simulink model "AC_Test"  (R2021b)
settings: Solver=VariableStepAuto  StartTime=0.0  StopTime=1  RelTol=1e-3
undefined symbols (not defined in the file): ac
libraries: fl_lib x132, nesl_utility x4
settings Model: Creator=김웅지  LastModifiedBy=김웅지

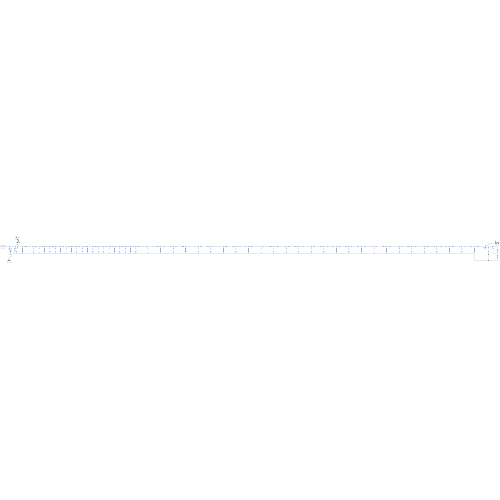
[thumbnail: Simulink's stored preview of the top-level diagram]
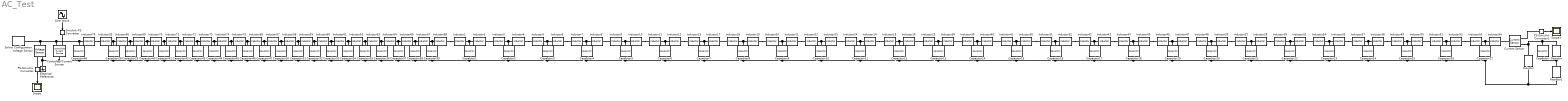
== system AC_Test ==
  Capacitor : fl_lib/Electrical/Electrical Elements/Capacitor  c=ac.rad.Cm1 F  r=1e-15 Ohm  g=0 1/Ohm  i_specify=off  i_priority=None  i=0 A  i_nominal_specify=off  i_nominal_unit=A  i_nominal_value=1  v_specify=off  v_priority=None  v=0 V  v_nominal_specify=off  v_nominal_unit=V  v_nominal_value=1  vc_specify=off  vc_priority=High  vc=0 V  vc_nominal_specify=off  vc_nominal_unit=V  vc_nominal_value=1
  Capacitor1 : fl_lib/Electrical/Electrical Elements/Capacitor  c=ac.ho.C(1) F  r=1e-15 Ohm  g=0 1/Ohm  i_specify=off  i_priority=None  i=0 A  i_nominal_specify=off  i_nominal_unit=A  i_nominal_value=1  v_specify=off  v_priority=None  v=0 V  v_nominal_specify=off  v_nominal_unit=V  v_nominal_value=1  vc_specify=off  vc_priority=High  vc=0 V  vc_nominal_specify=off  vc_nominal_unit=V  vc_nominal_value=1
  Capacitor10 : fl_lib/Electrical/Electrical Elements/Capacitor  c=ac.ho.C(10) F  r=1e-15 Ohm  g=0 1/Ohm  i_specify=off  i_priority=None  i=0 A  i_nominal_specify=off  i_nominal_unit=A  i_nominal_value=1  v_specify=off  v_priority=None  v=0 V  v_nominal_specify=off  v_nominal_unit=V  v_nominal_value=1  vc_specify=off  vc_priority=High  vc=0 V  vc_nominal_specify=off  vc_nominal_unit=V  vc_nominal_value=1
  Capacitor11 : fl_lib/Electrical/Electrical Elements/Capacitor  c=ac.ho.C(11) F  r=1e-15 Ohm  g=0 1/Ohm  i_specify=off  i_priority=None  i=0 A  i_nominal_specify=off  i_nominal_unit=A  i_nominal_value=1  v_specify=off  v_priority=None  v=0 V  v_nominal_specify=off  v_nominal_unit=V  v_nominal_value=1  vc_specify=off  vc_priority=High  vc=0 V  vc_nominal_specify=off  vc_nominal_unit=V  vc_nominal_value=1
  Capacitor12 : fl_lib/Electrical/Electrical Elements/Capacitor  c=ac.ho.C(12) F  r=1e-15 Ohm  g=0 1/Ohm  i_specify=off  i_priority=None  i=0 A  i_nominal_specify=off  i_nominal_unit=A  i_nominal_value=1  v_specify=off  v_priority=None  v=0 V  v_nominal_specify=off  v_nominal_unit=V  v_nominal_value=1  vc_specify=off  vc_priority=High  vc=0 V  vc_nominal_specify=off  vc_nominal_unit=V  vc_nominal_value=1
  Capacitor13 : fl_lib/Electrical/Electrical Elements/Capacitor  c=ac.ho.C(13) F  r=1e-15 Ohm  g=0 1/Ohm  i_specify=off  i_priority=None  i=0 A  i_nominal_specify=off  i_nominal_unit=A  i_nominal_value=1  v_specify=off  v_priority=None  v=0 V  v_nominal_specify=off  v_nominal_unit=V  v_nominal_value=1  vc_specify=off  vc_priority=High  vc=0 V  vc_nominal_specify=off  vc_nominal_unit=V  vc_nominal_value=1
  Capacitor14 : fl_lib/Electrical/Electrical Elements/Capacitor  c=ac.ho.C(14) F  r=1e-15 Ohm  g=0 1/Ohm  i_specify=off  i_priority=None  i=0 A  i_nominal_specify=off  i_nominal_unit=A  i_nominal_value=1  v_specify=off  v_priority=None  v=0 V  v_nominal_specify=off  v_nominal_unit=V  v_nominal_value=1  vc_specify=off  vc_priority=High  vc=0 V  vc_nominal_specify=off  vc_nominal_unit=V  vc_nominal_value=1
  Capacitor15 : fl_lib/Electrical/Electrical Elements/Capacitor  c=ac.ho.C(15) F  r=1e-15 Ohm  g=0 1/Ohm  i_specify=off  i_priority=None  i=0 A  i_nominal_specify=off  i_nominal_unit=A  i_nominal_value=1  v_specify=off  v_priority=None  v=0 V  v_nominal_specify=off  v_nominal_unit=V  v_nominal_value=1  vc_specify=off  vc_priority=High  vc=0 V  vc_nominal_specify=off  vc_nominal_unit=V  vc_nominal_value=1
  Capacitor16 : fl_lib/Electrical/Electrical Elements/Capacitor  c=ac.ho.C(16) F  r=1e-15 Ohm  g=0 1/Ohm  i_specify=off  i_priority=None  i=0 A  i_nominal_specify=off  i_nominal_unit=A  i_nominal_value=1  v_specify=off  v_priority=None  v=0 V  v_nominal_specify=off  v_nominal_unit=V  v_nominal_value=1  vc_specify=off  vc_priority=High  vc=0 V  vc_nominal_specify=off  vc_nominal_unit=V  vc_nominal_value=1
  Capacitor17 : fl_lib/Electrical/Electrical Elements/Capacitor  c=ac.ho.C(17) F  r=1e-15 Ohm  g=0 1/Ohm  i_specify=off  i_priority=None  i=0 A  i_nominal_specify=off  i_nominal_unit=A  i_nominal_value=1  v_specify=off  v_priority=None  v=0 V  v_nominal_specify=off  v_nominal_unit=V  v_nominal_value=1  vc_specify=off  vc_priority=High  vc=0 V  vc_nominal_specify=off  vc_nominal_unit=V  vc_nominal_value=1
  Capacitor18 : fl_lib/Electrical/Electrical Elements/Capacitor  c=ac.ho.C(18) F  r=1e-15 Ohm  g=0 1/Ohm  i_specify=off  i_priority=None  i=0 A  i_nominal_specify=off  i_nominal_unit=A  i_nominal_value=1  v_specify=off  v_priority=None  v=0 V  v_nominal_specify=off  v_nominal_unit=V  v_nominal_value=1  vc_specify=off  vc_priority=High  vc=0 V  vc_nominal_specify=off  vc_nominal_unit=V  vc_nominal_value=1
  Capacitor19 : fl_lib/Electrical/Electrical Elements/Capacitor  c=ac.ho.C(19) F  r=1e-15 Ohm  g=0 1/Ohm  i_specify=off  i_priority=None  i=0 A  i_nominal_specify=off  i_nominal_unit=A  i_nominal_value=1  v_specify=off  v_priority=None  v=0 V  v_nominal_specify=off  v_nominal_unit=V  v_nominal_value=1  vc_specify=off  vc_priority=High  vc=0 V  vc_nominal_specify=off  vc_nominal_unit=V  vc_nominal_value=1
  Capacitor2 : fl_lib/Electrical/Electrical Elements/Capacitor  c=ac.ho.C(2) F  r=1e-15 Ohm  g=0 1/Ohm  i_specify=off  i_priority=None  i=0 A  i_nominal_specify=off  i_nominal_unit=A  i_nominal_value=1  v_specify=off  v_priority=None  v=0 V  v_nominal_specify=off  v_nominal_unit=V  v_nominal_value=1  vc_specify=off  vc_priority=High  vc=0 V  vc_nominal_specify=off  vc_nominal_unit=V  vc_nominal_value=1
  Capacitor20 : fl_lib/Electrical/Electrical Elements/Capacitor  c=ac.ho.C(20) F  r=1e-15 Ohm  g=0 1/Ohm  i_specify=off  i_priority=None  i=0 A  i_nominal_specify=off  i_nominal_unit=A  i_nominal_value=1  v_specify=off  v_priority=None  v=0 V  v_nominal_specify=off  v_nominal_unit=V  v_nominal_value=1  vc_specify=off  vc_priority=High  vc=0 V  vc_nominal_specify=off  vc_nominal_unit=V  vc_nominal_value=1
  Capacitor21 : fl_lib/Electrical/Electrical Elements/Capacitor  c=ac.ho.C(21) F  r=1e-15 Ohm  g=0 1/Ohm  i_specify=off  i_priority=None  i=0 A  i_nominal_specify=off  i_nominal_unit=A  i_nominal_value=1  v_specify=off  v_priority=None  v=0 V  v_nominal_specify=off  v_nominal_unit=V  v_nominal_value=1  vc_specify=off  vc_priority=High  vc=0 V  vc_nominal_specify=off  vc_nominal_unit=V  vc_nominal_value=1
  Capacitor22 : fl_lib/Electrical/Electrical Elements/Capacitor  c=ac.ho.C(22) F  r=1e-15 Ohm  g=0 1/Ohm  i_specify=off  i_priority=None  i=0 A  i_nominal_specify=off  i_nominal_unit=A  i_nominal_value=1  v_specify=off  v_priority=None  v=0 V  v_nominal_specify=off  v_nominal_unit=V  v_nominal_value=1  vc_specify=off  vc_priority=High  vc=0 V  vc_nominal_specify=off  vc_nominal_unit=V  vc_nominal_value=1
  Capacitor23 : fl_lib/Electrical/Electrical Elements/Capacitor  c=ac.ho.C(23) F  r=1e-15 Ohm  g=0 1/Ohm  i_specify=off  i_priority=None  i=0 A  i_nominal_specify=off  i_nominal_unit=A  i_nominal_value=1  v_specify=off  v_priority=None  v=0 V  v_nominal_specify=off  v_nominal_unit=V  v_nominal_value=1  vc_specify=off  vc_priority=High  vc=0 V  vc_nominal_specify=off  vc_nominal_unit=V  vc_nominal_value=1
  Capacitor24 : fl_lib/Electrical/Electrical Elements/Capacitor  c=ac.ho.C(24) F  r=1e-15 Ohm  g=0 1/Ohm  i_specify=off  i_priority=None  i=0 A  i_nominal_specify=off  i_nominal_unit=A  i_nominal_value=1  v_specify=off  v_priority=None  v=0 V  v_nominal_specify=off  v_nominal_unit=V  v_nominal_value=1  vc_specify=off  vc_priority=High  vc=0 V  vc_nominal_specify=off  vc_nominal_unit=V  vc_nominal_value=1
  Capacitor25 : fl_lib/Electrical/Electrical Elements/Capacitor  c=ac.ho.C(25) F  r=1e-15 Ohm  g=0 1/Ohm  i_specify=off  i_priority=None  i=0 A  i_nominal_specify=off  i_nominal_unit=A  i_nominal_value=1  v_specify=off  v_priority=None  v=0 V  v_nominal_specify=off  v_nominal_unit=V  v_nominal_value=1  vc_specify=off  vc_priority=High  vc=0 V  vc_nominal_specify=off  vc_nominal_unit=V  vc_nominal_value=1
  Capacitor26 : fl_lib/Electrical/Electrical Elements/Capacitor  c=ac.ho.C(26) F  r=1e-15 Ohm  g=0 1/Ohm  i_specify=off  i_priority=None  i=0 A  i_nominal_specify=off  i_nominal_unit=A  i_nominal_value=1  v_specify=off  v_priority=None  v=0 V  v_nominal_specify=off  v_nominal_unit=V  v_nominal_value=1  vc_specify=off  vc_priority=High  vc=0 V  vc_nominal_specify=off  vc_nominal_unit=V  vc_nominal_value=1
  Capacitor27 : fl_lib/Electrical/Electrical Elements/Capacitor  c=ac.ho.C(27) F  r=1e-15 Ohm  g=0 1/Ohm  i_specify=off  i_priority=None  i=0 A  i_nominal_specify=off  i_nominal_unit=A  i_nominal_value=1  v_specify=off  v_priority=None  v=0 V  v_nominal_specify=off  v_nominal_unit=V  v_nominal_value=1  vc_specify=off  vc_priority=High  vc=0 V  vc_nominal_specify=off  vc_nominal_unit=V  vc_nominal_value=1
  Capacitor{28..47} (20 alike) : fl_lib/Electrical/Electrical Elements/Capacitor  c=ac.ps.C F  r=1e-15 Ohm  g=0 1/Ohm  i_specify=off  i_priority=None  i=0 A  i_nominal_specify=off  i_nominal_unit=A  i_nominal_value=1  v_specify=off  v_priority=None  v=0 V  v_nominal_specify=off  v_nominal_unit=V  v_nominal_value=1  vc_specify=off  vc_priority=High  vc=0 V  vc_nominal_specify=off  vc_nominal_unit=V  vc_nominal_value=1
  Capacitor3 : fl_lib/Electrical/Electrical Elements/Capacitor  c=ac.ho.C(3) F  r=1e-15 Ohm  g=0 1/Ohm  i_specify=off  i_priority=None  i=0 A  i_nominal_specify=off  i_nominal_unit=A  i_nominal_value=1  v_specify=off  v_priority=None  v=0 V  v_nominal_specify=off  v_nominal_unit=V  v_nominal_value=1  vc_specify=off  vc_priority=High  vc=0 V  vc_nominal_specify=off  vc_nominal_unit=V  vc_nominal_value=1
  Capacitor4 : fl_lib/Electrical/Electrical Elements/Capacitor  c=ac.ho.C(4) F  r=1e-15 Ohm  g=0 1/Ohm  i_specify=off  i_priority=None  i=0 A  i_nominal_specify=off  i_nominal_unit=A  i_nominal_value=1  v_specify=off  v_priority=None  v=0 V  v_nominal_specify=off  v_nominal_unit=V  v_nominal_value=1  vc_specify=off  vc_priority=High  vc=0 V  vc_nominal_specify=off  vc_nominal_unit=V  vc_nominal_value=1
  Capacitor48 : fl_lib/Electrical/Electrical Elements/Capacitor  c=ac.co.C F  r=1e-15 Ohm  g=0 1/Ohm  i_specify=off  i_priority=None  i=0 A  i_nominal_specify=off  i_nominal_unit=A  i_nominal_value=1  v_specify=off  v_priority=None  v=0 V  v_nominal_specify=off  v_nominal_unit=V  v_nominal_value=1  vc_specify=off  vc_priority=High  vc=0 V  vc_nominal_specify=off  vc_nominal_unit=V  vc_nominal_value=1
  Capacitor5 : fl_lib/Electrical/Electrical Elements/Capacitor  c=ac.ho.C(5) F  r=1e-15 Ohm  g=0 1/Ohm  i_specify=off  i_priority=None  i=0 A  i_nominal_specify=off  i_nominal_unit=A  i_nominal_value=1  v_specify=off  v_priority=None  v=0 V  v_nominal_specify=off  v_nominal_unit=V  v_nominal_value=1  vc_specify=off  vc_priority=High  vc=0 V  vc_nominal_specify=off  vc_nominal_unit=V  vc_nominal_value=1
  Capacitor6 : fl_lib/Electrical/Electrical Elements/Capacitor  c=ac.ho.C(6) F  r=1e-15 Ohm  g=0 1/Ohm  i_specify=off  i_priority=None  i=0 A  i_nominal_specify=off  i_nominal_unit=A  i_nominal_value=1  v_specify=off  v_priority=None  v=0 V  v_nominal_specify=off  v_nominal_unit=V  v_nominal_value=1  vc_specify=off  vc_priority=High  vc=0 V  vc_nominal_specify=off  vc_nominal_unit=V  vc_nominal_value=1
  Capacitor7 : fl_lib/Electrical/Electrical Elements/Capacitor  c=ac.ho.C(7) F  r=1e-15 Ohm  g=0 1/Ohm  i_specify=off  i_priority=None  i=0 A  i_nominal_specify=off  i_nominal_unit=A  i_nominal_value=1  v_specify=off  v_priority=None  v=0 V  v_nominal_specify=off  v_nominal_unit=V  v_nominal_value=1  vc_specify=off  vc_priority=High  vc=0 V  vc_nominal_specify=off  vc_nominal_unit=V  vc_nominal_value=1
  Capacitor8 : fl_lib/Electrical/Electrical Elements/Capacitor  c=ac.ho.C(8) F  r=1e-15 Ohm  g=0 1/Ohm  i_specify=off  i_priority=None  i=0 A  i_nominal_specify=off  i_nominal_unit=A  i_nominal_value=1  v_specify=off  v_priority=None  v=0 V  v_nominal_specify=off  v_nominal_unit=V  v_nominal_value=1  vc_specify=off  vc_priority=High  vc=0 V  vc_nominal_specify=off  vc_nominal_unit=V  vc_nominal_value=1
  Capacitor9 : fl_lib/Electrical/Electrical Elements/Capacitor  c=ac.ho.C(9) F  r=1e-15 Ohm  g=0 1/Ohm  i_specify=off  i_priority=None  i=0 A  i_nominal_specify=off  i_nominal_unit=A  i_nominal_value=1  v_specify=off  v_priority=None  v=0 V  v_nominal_specify=off  v_nominal_unit=V  v_nominal_value=1  vc_specify=off  vc_priority=High  vc=0 V  vc_nominal_specify=off  vc_nominal_unit=V  vc_nominal_value=1
  Controlled Current Source : fl_lib/Electrical/Electrical Sources/Controlled Current Source
  Current Sensor : fl_lib/Electrical/Electrical Sensors/Current Sensor
  Electrical Reference : fl_lib/Electrical/Electrical Elements/Electrical Reference
  Inductor : fl_lib/Electrical/Electrical Elements/Inductor  l=ac.rad.Mm1 H  r=0 Ohm  g=1e-15 1/Ohm  i_specify=off  i_priority=None  i=0 A  i_nominal_specify=off  i_nominal_unit=A  i_nominal_value=1  v_specify=off  v_priority=None  v=0 V  v_nominal_specify=off  v_nominal_unit=V  v_nominal_value=1  i_L_specify=off  i_L_priority=High  i_L=0 A  i_L_nominal_specify=off  i_L_nominal_unit=A  i_L_nominal_value=1
  Inductor1 : fl_lib/Electrical/Electrical Elements/Inductor  l=ac.ho.L(1) H  r=0 Ohm  g=1e-15 1/Ohm  i_specify=off  i_priority=None  i=0 A  i_nominal_specify=off  i_nominal_unit=A  i_nominal_value=1  v_specify=off  v_priority=None  v=0 V  v_nominal_specify=off  v_nominal_unit=V  v_nominal_value=1  i_L_specify=off  i_L_priority=High  i_L=0 A  i_L_nominal_specify=off  i_L_nominal_unit=A  i_L_nominal_value=1
  Inductor10 : fl_lib/Electrical/Electrical Elements/Inductor  l=ac.ho.L(5) H  r=0 Ohm  g=1e-15 1/Ohm  i_specify=off  i_priority=None  i=0 A  i_nominal_specify=off  i_nominal_unit=A  i_nominal_value=1  v_specify=off  v_priority=None  v=0 V  v_nominal_specify=off  v_nominal_unit=V  v_nominal_value=1  i_L_specify=off  i_L_priority=High  i_L=0 A  i_L_nominal_specify=off  i_L_nominal_unit=A  i_L_nominal_value=1
  Inductor11 : fl_lib/Electrical/Electrical Elements/Inductor  l=ac.ho.L(6) H  r=0 Ohm  g=1e-15 1/Ohm  i_specify=off  i_priority=None  i=0 A  i_nominal_specify=off  i_nominal_unit=A  i_nominal_value=1  v_specify=off  v_priority=None  v=0 V  v_nominal_specify=off  v_nominal_unit=V  v_nominal_value=1  i_L_specify=off  i_L_priority=High  i_L=0 A  i_L_nominal_specify=off  i_L_nominal_unit=A  i_L_nominal_value=1
  Inductor12 : fl_lib/Electrical/Electrical Elements/Inductor  l=ac.ho.L(6) H  r=0 Ohm  g=1e-15 1/Ohm  i_specify=off  i_priority=None  i=0 A  i_nominal_specify=off  i_nominal_unit=A  i_nominal_value=1  v_specify=off  v_priority=None  v=0 V  v_nominal_specify=off  v_nominal_unit=V  v_nominal_value=1  i_L_specify=off  i_L_priority=High  i_L=0 A  i_L_nominal_specify=off  i_L_nominal_unit=A  i_L_nominal_value=1
  Inductor13 : fl_lib/Electrical/Electrical Elements/Inductor  l=ac.ho.L(7) H  r=0 Ohm  g=1e-15 1/Ohm  i_specify=off  i_priority=None  i=0 A  i_nominal_specify=off  i_nominal_unit=A  i_nominal_value=1  v_specify=off  v_priority=None  v=0 V  v_nominal_specify=off  v_nominal_unit=V  v_nominal_value=1  i_L_specify=off  i_L_priority=High  i_L=0 A  i_L_nominal_specify=off  i_L_nominal_unit=A  i_L_nominal_value=1
  Inductor14 : fl_lib/Electrical/Electrical Elements/Inductor  l=ac.ho.L(11) H  r=0 Ohm  g=1e-15 1/Ohm  i_specify=off  i_priority=None  i=0 A  i_nominal_specify=off  i_nominal_unit=A  i_nominal_value=1  v_specify=off  v_priority=None  v=0 V  v_nominal_specify=off  v_nominal_unit=V  v_nominal_value=1  i_L_specify=off  i_L_priority=High  i_L=0 A  i_L_nominal_specify=off  i_L_nominal_unit=A  i_L_nominal_value=1
  Inductor15 : fl_lib/Electrical/Electrical Elements/Inductor  l=ac.ho.L(12) H  r=0 Ohm  g=1e-15 1/Ohm  i_specify=off  i_priority=None  i=0 A  i_nominal_specify=off  i_nominal_unit=A  i_nominal_value=1  v_specify=off  v_priority=None  v=0 V  v_nominal_specify=off  v_nominal_unit=V  v_nominal_value=1  i_L_specify=off  i_L_priority=High  i_L=0 A  i_L_nominal_specify=off  i_L_nominal_unit=A  i_L_nominal_value=1
  Inductor16 : fl_lib/Electrical/Electrical Elements/Inductor  l=ac.ho.L(12) H  r=0 Ohm  g=1e-15 1/Ohm  i_specify=off  i_priority=None  i=0 A  i_nominal_specify=off  i_nominal_unit=A  i_nominal_value=1  v_specify=off  v_priority=None  v=0 V  v_nominal_specify=off  v_nominal_unit=V  v_nominal_value=1  i_L_specify=off  i_L_priority=High  i_L=0 A  i_L_nominal_specify=off  i_L_nominal_unit=A  i_L_nominal_value=1
  Inductor17 : fl_lib/Electrical/Electrical Elements/Inductor  l=ac.ho.L(7) H  r=0 Ohm  g=1e-15 1/Ohm  i_specify=off  i_priority=None  i=0 A  i_nominal_specify=off  i_nominal_unit=A  i_nominal_value=1  v_specify=off  v_priority=None  v=0 V  v_nominal_specify=off  v_nominal_unit=V  v_nominal_value=1  i_L_specify=off  i_L_priority=High  i_L=0 A  i_L_nominal_specify=off  i_L_nominal_unit=A  i_L_nominal_value=1
  Inductor18 : fl_lib/Electrical/Electrical Elements/Inductor  l=ac.ho.L(8) H  r=0 Ohm  g=1e-15 1/Ohm  i_specify=off  i_priority=None  i=0 A  i_nominal_specify=off  i_nominal_unit=A  i_nominal_value=1  v_specify=off  v_priority=None  v=0 V  v_nominal_specify=off  v_nominal_unit=V  v_nominal_value=1  i_L_specify=off  i_L_priority=High  i_L=0 A  i_L_nominal_specify=off  i_L_nominal_unit=A  i_L_nominal_value=1
  Inductor19 : fl_lib/Electrical/Electrical Elements/Inductor  l=ac.ho.L(8) H  r=0 Ohm  g=1e-15 1/Ohm  i_specify=off  i_priority=None  i=0 A  i_nominal_specify=off  i_nominal_unit=A  i_nominal_value=1  v_specify=off  v_priority=None  v=0 V  v_nominal_specify=off  v_nominal_unit=V  v_nominal_value=1  i_L_specify=off  i_L_priority=High  i_L=0 A  i_L_nominal_specify=off  i_L_nominal_unit=A  i_L_nominal_value=1
  Inductor2 : fl_lib/Electrical/Electrical Elements/Inductor  l=ac.ho.L(1) H  r=0 Ohm  g=1e-15 1/Ohm  i_specify=off  i_priority=None  i=0 A  i_nominal_specify=off  i_nominal_unit=A  i_nominal_value=1  v_specify=off  v_priority=None  v=0 V  v_nominal_specify=off  v_nominal_unit=V  v_nominal_value=1  i_L_specify=off  i_L_priority=High  i_L=0 A  i_L_nominal_specify=off  i_L_nominal_unit=A  i_L_nominal_value=1
  Inductor20 : fl_lib/Electrical/Electrical Elements/Inductor  l=ac.ho.L(9) H  r=0 Ohm  g=1e-15 1/Ohm  i_specify=off  i_priority=None  i=0 A  i_nominal_specify=off  i_nominal_unit=A  i_nominal_value=1  v_specify=off  v_priority=None  v=0 V  v_nominal_specify=off  v_nominal_unit=V  v_nominal_value=1  i_L_specify=off  i_L_priority=High  i_L=0 A  i_L_nominal_specify=off  i_L_nominal_unit=A  i_L_nominal_value=1
  Inductor21 : fl_lib/Electrical/Electrical Elements/Inductor  l=ac.ho.L(9) H  r=0 Ohm  g=1e-15 1/Ohm  i_specify=off  i_priority=None  i=0 A  i_nominal_specify=off  i_nominal_unit=A  i_nominal_value=1  v_specify=off  v_priority=None  v=0 V  v_nominal_specify=off  v_nominal_unit=V  v_nominal_value=1  i_L_specify=off  i_L_priority=High  i_L=0 A  i_L_nominal_specify=off  i_L_nominal_unit=A  i_L_nominal_value=1
  Inductor22 : fl_lib/Electrical/Electrical Elements/Inductor  l=ac.ho.L(10) H  r=0 Ohm  g=1e-15 1/Ohm  i_specify=off  i_priority=None  i=0 A  i_nominal_specify=off  i_nominal_unit=A  i_nominal_value=1  v_specify=off  v_priority=None  v=0 V  v_nominal_specify=off  v_nominal_unit=V  v_nominal_value=1  i_L_specify=off  i_L_priority=High  i_L=0 A  i_L_nominal_specify=off  i_L_nominal_unit=A  i_L_nominal_value=1
  Inductor23 : fl_lib/Electrical/Electrical Elements/Inductor  l=ac.ho.L(10) H  r=0 Ohm  g=1e-15 1/Ohm  i_specify=off  i_priority=None  i=0 A  i_nominal_specify=off  i_nominal_unit=A  i_nominal_value=1  v_specify=off  v_priority=None  v=0 V  v_nominal_specify=off  v_nominal_unit=V  v_nominal_value=1  i_L_specify=off  i_L_priority=High  i_L=0 A  i_L_nominal_specify=off  i_L_nominal_unit=A  i_L_nominal_value=1
  Inductor24 : fl_lib/Electrical/Electrical Elements/Inductor  l=ac.ho.L(11) H  r=0 Ohm  g=1e-15 1/Ohm  i_specify=off  i_priority=None  i=0 A  i_nominal_specify=off  i_nominal_unit=A  i_nominal_value=1  v_specify=off  v_priority=None  v=0 V  v_nominal_specify=off  v_nominal_unit=V  v_nominal_value=1  i_L_specify=off  i_L_priority=High  i_L=0 A  i_L_nominal_specify=off  i_L_nominal_unit=A  i_L_nominal_value=1
  Inductor25 : fl_lib/Electrical/Electrical Elements/Inductor  l=ac.ho.L(13) H  r=0 Ohm  g=1e-15 1/Ohm  i_specify=off  i_priority=None  i=0 A  i_nominal_specify=off  i_nominal_unit=A  i_nominal_value=1  v_specify=off  v_priority=None  v=0 V  v_nominal_specify=off  v_nominal_unit=V  v_nominal_value=1  i_L_specify=off  i_L_priority=High  i_L=0 A  i_L_nominal_specify=off  i_L_nominal_unit=A  i_L_nominal_value=1
  Inductor26 : fl_lib/Electrical/Electrical Elements/Inductor  l=ac.ho.L(20) H  r=0 Ohm  g=1e-15 1/Ohm  i_specify=off  i_priority=None  i=0 A  i_nominal_specify=off  i_nominal_unit=A  i_nominal_value=1  v_specify=off  v_priority=None  v=0 V  v_nominal_specify=off  v_nominal_unit=V  v_nominal_value=1  i_L_specify=off  i_L_priority=High  i_L=0 A  i_L_nominal_specify=off  i_L_nominal_unit=A  i_L_nominal_value=1
  Inductor27 : fl_lib/Electrical/Electrical Elements/Inductor  l=ac.ho.L(21) H  r=0 Ohm  g=1e-15 1/Ohm  i_specify=off  i_priority=None  i=0 A  i_nominal_specify=off  i_nominal_unit=A  i_nominal_value=1  v_specify=off  v_priority=None  v=0 V  v_nominal_specify=off  v_nominal_unit=V  v_nominal_value=1  i_L_specify=off  i_L_priority=High  i_L=0 A  i_L_nominal_specify=off  i_L_nominal_unit=A  i_L_nominal_value=1
  Inductor28 : fl_lib/Electrical/Electrical Elements/Inductor  l=ac.ho.L(21) H  r=0 Ohm  g=1e-15 1/Ohm  i_specify=off  i_priority=None  i=0 A  i_nominal_specify=off  i_nominal_unit=A  i_nominal_value=1  v_specify=off  v_priority=None  v=0 V  v_nominal_specify=off  v_nominal_unit=V  v_nominal_value=1  i_L_specify=off  i_L_priority=High  i_L=0 A  i_L_nominal_specify=off  i_L_nominal_unit=A  i_L_nominal_value=1
  Inductor29 : fl_lib/Electrical/Electrical Elements/Inductor  l=ac.ho.L(22) H  r=0 Ohm  g=1e-15 1/Ohm  i_specify=off  i_priority=None  i=0 A  i_nominal_specify=off  i_nominal_unit=A  i_nominal_value=1  v_specify=off  v_priority=None  v=0 V  v_nominal_specify=off  v_nominal_unit=V  v_nominal_value=1  i_L_specify=off  i_L_priority=High  i_L=0 A  i_L_nominal_specify=off  i_L_nominal_unit=A  i_L_nominal_value=1
  Inductor3 : fl_lib/Electrical/Electrical Elements/Inductor  l=ac.ho.L(2) H  r=0 Ohm  g=1e-15 1/Ohm  i_specify=off  i_priority=None  i=0 A  i_nominal_specify=off  i_nominal_unit=A  i_nominal_value=1  v_specify=off  v_priority=None  v=0 V  v_nominal_specify=off  v_nominal_unit=V  v_nominal_value=1  i_L_specify=off  i_L_priority=High  i_L=0 A  i_L_nominal_specify=off  i_L_nominal_unit=A  i_L_nominal_value=1
  Inductor30 : fl_lib/Electrical/Electrical Elements/Inductor  l=ac.ho.L(15) H  r=0 Ohm  g=1e-15 1/Ohm  i_specify=off  i_priority=None  i=0 A  i_nominal_specify=off  i_nominal_unit=A  i_nominal_value=1  v_specify=off  v_priority=None  v=0 V  v_nominal_specify=off  v_nominal_unit=V  v_nominal_value=1  i_L_specify=off  i_L_priority=High  i_L=0 A  i_L_nominal_specify=off  i_L_nominal_unit=A  i_L_nominal_value=1
  Inductor31 : fl_lib/Electrical/Electrical Elements/Inductor  l=ac.ho.L(16) H  r=0 Ohm  g=1e-15 1/Ohm  i_specify=off  i_priority=None  i=0 A  i_nominal_specify=off  i_nominal_unit=A  i_nominal_value=1  v_specify=off  v_priority=None  v=0 V  v_nominal_specify=off  v_nominal_unit=V  v_nominal_value=1  i_L_specify=off  i_L_priority=High  i_L=0 A  i_L_nominal_specify=off  i_L_nominal_unit=A  i_L_nominal_value=1
  Inductor32 : fl_lib/Electrical/Electrical Elements/Inductor  l=ac.ho.L(16) H  r=0 Ohm  g=1e-15 1/Ohm  i_specify=off  i_priority=None  i=0 A  i_nominal_specify=off  i_nominal_unit=A  i_nominal_value=1  v_specify=off  v_priority=None  v=0 V  v_nominal_specify=off  v_nominal_unit=V  v_nominal_value=1  i_L_specify=off  i_L_priority=High  i_L=0 A  i_L_nominal_specify=off  i_L_nominal_unit=A  i_L_nominal_value=1
  Inductor33 : fl_lib/Electrical/Electrical Elements/Inductor  l=ac.ho.L(22) H  r=0 Ohm  g=1e-15 1/Ohm  i_specify=off  i_priority=None  i=0 A  i_nominal_specify=off  i_nominal_unit=A  i_nominal_value=1  v_specify=off  v_priority=None  v=0 V  v_nominal_specify=off  v_nominal_unit=V  v_nominal_value=1  i_L_specify=off  i_L_priority=High  i_L=0 A  i_L_nominal_specify=off  i_L_nominal_unit=A  i_L_nominal_value=1
  Inductor34 : fl_lib/Electrical/Electrical Elements/Inductor  l=ac.ho.L(23) H  r=0 Ohm  g=1e-15 1/Ohm  i_specify=off  i_priority=None  i=0 A  i_nominal_specify=off  i_nominal_unit=A  i_nominal_value=1  v_specify=off  v_priority=None  v=0 V  v_nominal_specify=off  v_nominal_unit=V  v_nominal_value=1  i_L_specify=off  i_L_priority=High  i_L=0 A  i_L_nominal_specify=off  i_L_nominal_unit=A  i_L_nominal_value=1
  Inductor35 : fl_lib/Electrical/Electrical Elements/Inductor  l=ac.ho.L(23) H  r=0 Ohm  g=1e-15 1/Ohm  i_specify=off  i_priority=None  i=0 A  i_nominal_specify=off  i_nominal_unit=A  i_nominal_value=1  v_specify=off  v_priority=None  v=0 V  v_nominal_specify=off  v_nominal_unit=V  v_nominal_value=1  i_L_specify=off  i_L_priority=High  i_L=0 A  i_L_nominal_specify=off  i_L_nominal_unit=A  i_L_nominal_value=1
  Inductor36 : fl_lib/Electrical/Electrical Elements/Inductor  l=ac.ho.L(13) H  r=0 Ohm  g=1e-15 1/Ohm  i_specify=off  i_priority=None  i=0 A  i_nominal_specify=off  i_nominal_unit=A  i_nominal_value=1  v_specify=off  v_priority=None  v=0 V  v_nominal_specify=off  v_nominal_unit=V  v_nominal_value=1  i_L_specify=off  i_L_priority=High  i_L=0 A  i_L_nominal_specify=off  i_L_nominal_unit=A  i_L_nominal_value=1
  Inductor37 : fl_lib/Electrical/Electrical Elements/Inductor  l=ac.ho.L(24) H  r=0 Ohm  g=1e-15 1/Ohm  i_specify=off  i_priority=None  i=0 A  i_nominal_specify=off  i_nominal_unit=A  i_nominal_value=1  v_specify=off  v_priority=None  v=0 V  v_nominal_specify=off  v_nominal_unit=V  v_nominal_value=1  i_L_specify=off  i_L_priority=High  i_L=0 A  i_L_nominal_specify=off  i_L_nominal_unit=A  i_L_nominal_value=1
  Inductor38 : fl_lib/Electrical/Electrical Elements/Inductor  l=ac.ho.L(24) H  r=0 Ohm  g=1e-15 1/Ohm  i_specify=off  i_priority=None  i=0 A  i_nominal_specify=off  i_nominal_unit=A  i_nominal_value=1  v_specify=off  v_priority=None  v=0 V  v_nominal_specify=off  v_nominal_unit=V  v_nominal_value=1  i_L_specify=off  i_L_priority=High  i_L=0 A  i_L_nominal_specify=off  i_L_nominal_unit=A  i_L_nominal_value=1
  Inductor39 : fl_lib/Electrical/Electrical Elements/Inductor  l=ac.ho.L(14) H  r=0 Ohm  g=1e-15 1/Ohm  i_specify=off  i_priority=None  i=0 A  i_nominal_specify=off  i_nominal_unit=A  i_nominal_value=1  v_specify=off  v_priority=None  v=0 V  v_nominal_specify=off  v_nominal_unit=V  v_nominal_value=1  i_L_specify=off  i_L_priority=High  i_L=0 A  i_L_nominal_specify=off  i_L_nominal_unit=A  i_L_nominal_value=1
  Inductor4 : fl_lib/Electrical/Electrical Elements/Inductor  l=ac.ho.L(2) H  r=0 Ohm  g=1e-15 1/Ohm  i_specify=off  i_priority=None  i=0 A  i_nominal_specify=off  i_nominal_unit=A  i_nominal_value=1  v_specify=off  v_priority=None  v=0 V  v_nominal_specify=off  v_nominal_unit=V  v_nominal_value=1  i_L_specify=off  i_L_priority=High  i_L=0 A  i_L_nominal_specify=off  i_L_nominal_unit=A  i_L_nominal_value=1
  Inductor40 : fl_lib/Electrical/Electrical Elements/Inductor  l=ac.ho.L(14) H  r=0 Ohm  g=1e-15 1/Ohm  i_specify=off  i_priority=None  i=0 A  i_nominal_specify=off  i_nominal_unit=A  i_nominal_value=1  v_specify=off  v_priority=None  v=0 V  v_nominal_specify=off  v_nominal_unit=V  v_nominal_value=1  i_L_specify=off  i_L_priority=High  i_L=0 A  i_L_nominal_specify=off  i_L_nominal_unit=A  i_L_nominal_value=1
  Inductor41 : fl_lib/Electrical/Electrical Elements/Inductor  l=ac.ho.L(15) H  r=0 Ohm  g=1e-15 1/Ohm  i_specify=off  i_priority=None  i=0 A  i_nominal_specify=off  i_nominal_unit=A  i_nominal_value=1  v_specify=off  v_priority=None  v=0 V  v_nominal_specify=off  v_nominal_unit=V  v_nominal_value=1  i_L_specify=off  i_L_priority=High  i_L=0 A  i_L_nominal_specify=off  i_L_nominal_unit=A  i_L_nominal_value=1
  Inductor42 : fl_lib/Electrical/Electrical Elements/Inductor  l=ac.ho.L(17) H  r=0 Ohm  g=1e-15 1/Ohm  i_specify=off  i_priority=None  i=0 A  i_nominal_specify=off  i_nominal_unit=A  i_nominal_value=1  v_specify=off  v_priority=None  v=0 V  v_nominal_specify=off  v_nominal_unit=V  v_nominal_value=1  i_L_specify=off  i_L_priority=High  i_L=0 A  i_L_nominal_specify=off  i_L_nominal_unit=A  i_L_nominal_value=1
  Inductor43 : fl_lib/Electrical/Electrical Elements/Inductor  l=ac.ho.L(17) H  r=0 Ohm  g=1e-15 1/Ohm  i_specify=off  i_priority=None  i=0 A  i_nominal_specify=off  i_nominal_unit=A  i_nominal_value=1  v_specify=off  v_priority=None  v=0 V  v_nominal_specify=off  v_nominal_unit=V  v_nominal_value=1  i_L_specify=off  i_L_priority=High  i_L=0 A  i_L_nominal_specify=off  i_L_nominal_unit=A  i_L_nominal_value=1
  Inductor44 : fl_lib/Electrical/Electrical Elements/Inductor  l=ac.ho.L(18) H  r=0 Ohm  g=1e-15 1/Ohm  i_specify=off  i_priority=None  i=0 A  i_nominal_specify=off  i_nominal_unit=A  i_nominal_value=1  v_specify=off  v_priority=None  v=0 V  v_nominal_specify=off  v_nominal_unit=V  v_nominal_value=1  i_L_specify=off  i_L_priority=High  i_L=0 A  i_L_nominal_specify=off  i_L_nominal_unit=A  i_L_nominal_value=1
  Inductor45 : fl_lib/Electrical/Electrical Elements/Inductor  l=ac.ho.L(18) H  r=0 Ohm  g=1e-15 1/Ohm  i_specify=off  i_priority=None  i=0 A  i_nominal_specify=off  i_nominal_unit=A  i_nominal_value=1  v_specify=off  v_priority=None  v=0 V  v_nominal_specify=off  v_nominal_unit=V  v_nominal_value=1  i_L_specify=off  i_L_priority=High  i_L=0 A  i_L_nominal_specify=off  i_L_nominal_unit=A  i_L_nominal_value=1
  Inductor46 : fl_lib/Electrical/Electrical Elements/Inductor  l=ac.ho.L(19) H  r=0 Ohm  g=1e-15 1/Ohm  i_specify=off  i_priority=None  i=0 A  i_nominal_specify=off  i_nominal_unit=A  i_nominal_value=1  v_specify=off  v_priority=None  v=0 V  v_nominal_specify=off  v_nominal_unit=V  v_nominal_value=1  i_L_specify=off  i_L_priority=High  i_L=0 A  i_L_nominal_specify=off  i_L_nominal_unit=A  i_L_nominal_value=1
  Inductor47 : fl_lib/Electrical/Electrical Elements/Inductor  l=ac.ho.L(19) H  r=0 Ohm  g=1e-15 1/Ohm  i_specify=off  i_priority=None  i=0 A  i_nominal_specify=off  i_nominal_unit=A  i_nominal_value=1  v_specify=off  v_priority=None  v=0 V  v_nominal_specify=off  v_nominal_unit=V  v_nominal_value=1  i_L_specify=off  i_L_priority=High  i_L=0 A  i_L_nominal_specify=off  i_L_nominal_unit=A  i_L_nominal_value=1
  Inductor48 : fl_lib/Electrical/Electrical Elements/Inductor  l=ac.ho.L(20) H  r=0 Ohm  g=1e-15 1/Ohm  i_specify=off  i_priority=None  i=0 A  i_nominal_specify=off  i_nominal_unit=A  i_nominal_value=1  v_specify=off  v_priority=None  v=0 V  v_nominal_specify=off  v_nominal_unit=V  v_nominal_value=1  i_L_specify=off  i_L_priority=High  i_L=0 A  i_L_nominal_specify=off  i_L_nominal_unit=A  i_L_nominal_value=1
  Inductor49 : fl_lib/Electrical/Electrical Elements/Inductor  l=ac.ho.L(25) H  r=0 Ohm  g=1e-15 1/Ohm  i_specify=off  i_priority=None  i=0 A  i_nominal_specify=off  i_nominal_unit=A  i_nominal_value=1  v_specify=off  v_priority=None  v=0 V  v_nominal_specify=off  v_nominal_unit=V  v_nominal_value=1  i_L_specify=off  i_L_priority=High  i_L=0 A  i_L_nominal_specify=off  i_L_nominal_unit=A  i_L_nominal_value=1
  Inductor5 : fl_lib/Electrical/Electrical Elements/Inductor  l=ac.ho.L(3) H  r=0 Ohm  g=1e-15 1/Ohm  i_specify=off  i_priority=None  i=0 A  i_nominal_specify=off  i_nominal_unit=A  i_nominal_value=1  v_specify=off  v_priority=None  v=0 V  v_nominal_specify=off  v_nominal_unit=V  v_nominal_value=1  i_L_specify=off  i_L_priority=High  i_L=0 A  i_L_nominal_specify=off  i_L_nominal_unit=A  i_L_nominal_value=1
  Inductor50 : fl_lib/Electrical/Electrical Elements/Inductor  l=ac.ho.L(25) H  r=0 Ohm  g=1e-15 1/Ohm  i_specify=off  i_priority=None  i=0 A  i_nominal_specify=off  i_nominal_unit=A  i_nominal_value=1  v_specify=off  v_priority=None  v=0 V  v_nominal_specify=off  v_nominal_unit=V  v_nominal_value=1  i_L_specify=off  i_L_priority=High  i_L=0 A  i_L_nominal_specify=off  i_L_nominal_unit=A  i_L_nominal_value=1
  Inductor51 : fl_lib/Electrical/Electrical Elements/Inductor  l=ac.ho.L(26) H  r=0 Ohm  g=1e-15 1/Ohm  i_specify=off  i_priority=None  i=0 A  i_nominal_specify=off  i_nominal_unit=A  i_nominal_value=1  v_specify=off  v_priority=None  v=0 V  v_nominal_specify=off  v_nominal_unit=V  v_nominal_value=1  i_L_specify=off  i_L_priority=High  i_L=0 A  i_L_nominal_specify=off  i_L_nominal_unit=A  i_L_nominal_value=1
  Inductor52 : fl_lib/Electrical/Electrical Elements/Inductor  l=ac.ho.L(26) H  r=0 Ohm  g=1e-15 1/Ohm  i_specify=off  i_priority=None  i=0 A  i_nominal_specify=off  i_nominal_unit=A  i_nominal_value=1  v_specify=off  v_priority=None  v=0 V  v_nominal_specify=off  v_nominal_unit=V  v_nominal_value=1  i_L_specify=off  i_L_priority=High  i_L=0 A  i_L_nominal_specify=off  i_L_nominal_unit=A  i_L_nominal_value=1
  Inductor53 : fl_lib/Electrical/Electrical Elements/Inductor  l=ac.ho.L(27) H  r=0 Ohm  g=1e-15 1/Ohm  i_specify=off  i_priority=None  i=0 A  i_nominal_specify=off  i_nominal_unit=A  i_nominal_value=1  v_specify=off  v_priority=None  v=0 V  v_nominal_specify=off  v_nominal_unit=V  v_nominal_value=1  i_L_specify=off  i_L_priority=High  i_L=0 A  i_L_nominal_specify=off  i_L_nominal_unit=A  i_L_nominal_value=1
  Inductor54 : fl_lib/Electrical/Electrical Elements/Inductor  l=ac.ho.L(27) H  r=0 Ohm  g=1e-15 1/Ohm  i_specify=off  i_priority=None  i=0 A  i_nominal_specify=off  i_nominal_unit=A  i_nominal_value=1  v_specify=off  v_priority=None  v=0 V  v_nominal_specify=off  v_nominal_unit=V  v_nominal_value=1  i_L_specify=off  i_L_priority=High  i_L=0 A  i_L_nominal_specify=off  i_L_nominal_unit=A  i_L_nominal_value=1
  Inductor55 : fl_lib/Electrical/Electrical Elements/Inductor  l=ac.ps.L/2 H  r=0 Ohm  g=1e-15 1/Ohm  i_specify=off  i_priority=None  i=0 A  i_nominal_specify=off  i_nominal_unit=A  i_nominal_value=1  v_specify=off  v_priority=None  v=0 V  v_nominal_specify=off  v_nominal_unit=V  v_nominal_value=1  i_L_specify=off  i_L_priority=High  i_L=0 A  i_L_nominal_specify=off  i_L_nominal_unit=A  i_L_nominal_value=1
  Inductor{56..67,69..75} (19 alike) : fl_lib/Electrical/Electrical Elements/Inductor  l=ac.ps.L H  r=0 Ohm  g=1e-15 1/Ohm  i_specify=off  i_priority=None  i=0 A  i_nominal_specify=off  i_nominal_unit=A  i_nominal_value=1  v_specify=off  v_priority=None  v=0 V  v_nominal_specify=off  v_nominal_unit=V  v_nominal_value=1  i_L_specify=off  i_L_priority=High  i_L=0 A  i_L_nominal_specify=off  i_L_nominal_unit=A  i_L_nominal_value=1
  Inductor6 : fl_lib/Electrical/Electrical Elements/Inductor  l=ac.ho.L(3) H  r=0 Ohm  g=1e-15 1/Ohm  i_specify=off  i_priority=None  i=0 A  i_nominal_specify=off  i_nominal_unit=A  i_nominal_value=1  v_specify=off  v_priority=None  v=0 V  v_nominal_specify=off  v_nominal_unit=V  v_nominal_value=1  i_L_specify=off  i_L_priority=High  i_L=0 A  i_L_nominal_specify=off  i_L_nominal_unit=A  i_L_nominal_value=1
  Inductor68 : fl_lib/Electrical/Electrical Elements/Inductor  l=ac.ps.L/2 H  r=0 Ohm  g=1e-15 1/Ohm  i_specify=off  i_priority=None  i=0 A  i_nominal_specify=off  i_nominal_unit=A  i_nominal_value=1  v_specify=off  v_priority=None  v=0 V  v_nominal_specify=off  v_nominal_unit=V  v_nominal_value=1  i_L_specify=off  i_L_priority=High  i_L=0 A  i_L_nominal_specify=off  i_L_nominal_unit=A  i_L_nominal_value=1
  Inductor7 : fl_lib/Electrical/Electrical Elements/Inductor  l=ac.ho.L(4) H  r=0 Ohm  g=1e-15 1/Ohm  i_specify=off  i_priority=None  i=0 A  i_nominal_specify=off  i_nominal_unit=A  i_nominal_value=1  v_specify=off  v_priority=None  v=0 V  v_nominal_specify=off  v_nominal_unit=V  v_nominal_value=1  i_L_specify=off  i_L_priority=High  i_L=0 A  i_L_nominal_specify=off  i_L_nominal_unit=A  i_L_nominal_value=1
  Inductor76 : fl_lib/Electrical/Electrical Elements/Inductor  l=ac.co.L H  r=0 Ohm  g=1e-15 1/Ohm  i_specify=off  i_priority=None  i=0 A  i_nominal_specify=off  i_nominal_unit=A  i_nominal_value=1  v_specify=off  v_priority=None  v=0 V  v_nominal_specify=off  v_nominal_unit=V  v_nominal_value=1  i_L_specify=off  i_L_priority=High  i_L=0 A  i_L_nominal_specify=off  i_L_nominal_unit=A  i_L_nominal_value=1
  Inductor8 : fl_lib/Electrical/Electrical Elements/Inductor  l=ac.ho.L(4) H  r=0 Ohm  g=1e-15 1/Ohm  i_specify=off  i_priority=None  i=0 A  i_nominal_specify=off  i_nominal_unit=A  i_nominal_value=1  v_specify=off  v_priority=None  v=0 V  v_nominal_specify=off  v_nominal_unit=V  v_nominal_value=1  i_L_specify=off  i_L_priority=High  i_L=0 A  i_L_nominal_specify=off  i_L_nominal_unit=A  i_L_nominal_value=1
  Inductor9 : fl_lib/Electrical/Electrical Elements/Inductor  l=ac.ho.L(5) H  r=0 Ohm  g=1e-15 1/Ohm  i_specify=off  i_priority=None  i=0 A  i_nominal_specify=off  i_nominal_unit=A  i_nominal_value=1  v_specify=off  v_priority=None  v=0 V  v_nominal_specify=off  v_nominal_unit=V  v_nominal_value=1  i_L_specify=off  i_L_priority=High  i_L=0 A  i_L_nominal_specify=off  i_L_nominal_unit=A  i_L_nominal_value=1
  PS-Simulink Converter : nesl_utility/PS-Simulink Converter  PhysicalDomain=network_engine_domain  SubClassName=ps_output  LeftPortType=input  RightPortType=output  PseudoPeriodic=off  Frequencies=[]  Unit=inherit  AffineConversion=off
      settings: SourceProductBaseCode=PW,SS
  PS-Simulink Converter1 : nesl_utility/PS-Simulink Converter  PhysicalDomain=network_engine_domain  SubClassName=ps_output  LeftPortType=input  RightPortType=output  PseudoPeriodic=off  Frequencies=[]  Unit=inherit  AffineConversion=off
      settings: SourceProductBaseCode=PW,SS
  Resistor : fl_lib/Electrical/Electrical Elements/Resistor  R=ac.rad.Rm1 Ohm  i_specify=off  i_priority=None  i=0 A  i_nominal_specify=off  i_nominal_unit=A  i_nominal_value=1  v_specify=off  v_priority=None  v=0 V  v_nominal_specify=off  v_nominal_unit=V  v_nominal_value=1
  Resistor1 : fl_lib/Electrical/Electrical Elements/Resistor  R=ac.rad.Rm2 Ohm  i_specify=off  i_priority=None  i=0 A  i_nominal_specify=off  i_nominal_unit=A  i_nominal_value=1  v_specify=off  v_priority=None  v=0 V  v_nominal_specify=off  v_nominal_unit=V  v_nominal_value=1
  Scope : Scope
  Scope1 : Scope
  Simulink-PS Converter : nesl_utility/Simulink-PS Converter  PhysicalDomain=network_engine_domain  SubClassName=ps_input  LeftPortType=input  RightPortType=output  PseudoPeriodic=off  Frequencies=[]  NoiseDistribution=none  NoiseParameters=[]  Unit=1  AffineConversion=off  FilteringAndDerivatives=provide  SimscapeFilterOrder=1  InputFilterTimeConstant=0.001  UdotUserProvided=0
      settings: SourceProductBaseCode=PW,SS
  Sine Wave : Sin  Frequency=2*pi*1e3  SampleTime=0
  Solver Configuration : nesl_utility/Solver Configuration  PhysicalDomain=network_engine_domain  SubClassName=solver  LeftPortType=input  RightPortType=generic  Tones=[]  Harmonics=[]  SimulateNoise=off  Profile=off  UseLocalSampling=off  EnableSwitchedLinearOptims=on  FrequencyDomain=off  UseCCode=off  RelTol=0.001  AbsTol=1e-06  MinStep=1e-09  ToWorkspace=off  RevertToSquareIcSolve=off  NumHomotopyIterations=100  PhasorMode=off  PhasorModeNumHarmonics=1  DoDC=off  ResidualTolerance=1e-09  UseLocalSolver=off  LocalSolverChoice=NE_BACKWARD_EULER_ADVANCER  LocalSolverSampleTime=0.001  DoFixedCost=off  MaxNonlinIter=3  MaxModeIter=2  ComputeImpulses=off  ImpulseIterations=2  LinearAlgebra=auto  EquationFormulation=NE_TIME_EF  DelaysMemoryBudget=1024  AutomaticFiltering=on  FilteringTimeConstant=0.001  PartitionStorageMethod=AS_NEEDED  PartitionMemoryBudget=1024  PartitionMethod=ROBUST
      settings: SourceProductBaseCode=PW,SS
  Voltage Sensor : fl_lib/Electrical/Electrical Sensors/Voltage Sensor
  wires:
  PS-Simulink Converter/1 -> Scope/1
  Sine Wave/1 -> Simulink-PS Converter/1
  PS-Simulink Converter1/1 -> Scope1/1
  connections:
  Capacitor/LConn1 -- Current Sensor/RConn2 -- Inductor/LConn1 -- Resistor/LConn1
  Capacitor/RConn1 -- Resistor1/LConn1 -- Resistor/RConn1
  Inductor47/LConn1 -- Inductor46/RConn1 -- Capacitor19/LConn1
  Inductor36/LConn1 -- Inductor25/RConn1 -- Capacitor13/LConn1
  Inductor52/LConn1 -- Inductor51/RConn1 -- Capacitor26/LConn1
  Inductor45/LConn1 -- Inductor44/RConn1 -- Capacitor18/LConn1
  Inductor43/LConn1 -- Inductor42/RConn1 -- Capacitor17/LConn1
  Inductor35/LConn1 -- Inductor34/RConn1 -- Capacitor23/LConn1
  Inductor38/LConn1 -- Inductor37/RConn1 -- Capacitor24/LConn1
  Inductor40/LConn1 -- Inductor39/RConn1 -- Capacitor14/LConn1
  Inductor10/LConn1 -- Inductor9/RConn1 -- Capacitor5/LConn1
  Inductor17/LConn1 -- Inductor13/RConn1 -- Capacitor7/LConn1
  Inductor14/LConn1 -- Inductor24/RConn1 -- Capacitor11/LConn1
  Inductor19/LConn1 -- Inductor18/RConn1 -- Capacitor8/LConn1
  Inductor30/LConn1 -- Inductor41/RConn1 -- Capacitor15/LConn1
  Inductor33/LConn1 -- Inductor29/RConn1 -- Capacitor22/LConn1
  Inductor23/LConn1 -- Inductor22/RConn1 -- Capacitor10/LConn1
  Inductor8/LConn1 -- Inductor7/RConn1 -- Capacitor4/LConn1
  Inductor21/LConn1 -- Inductor20/RConn1 -- Capacitor9/LConn1
  Inductor32/LConn1 -- Inductor31/RConn1 -- Capacitor16/LConn1
  Inductor26/LConn1 -- Inductor48/RConn1 -- Capacitor20/LConn1
  Inductor2/LConn1 -- Inductor1/RConn1 -- Capacitor1/LConn1
  Inductor12/LConn1 -- Inductor11/RConn1 -- Capacitor6/LConn1
  Inductor4/LConn1 -- Inductor3/RConn1 -- Capacitor2/LConn1
  Inductor28/LConn1 -- Inductor27/RConn1 -- Capacitor21/LConn1
  Inductor6/LConn1 -- Inductor5/RConn1 -- Capacitor3/LConn1
  Inductor16/LConn1 -- Inductor15/RConn1 -- Capacitor12/LConn1
  Inductor50/LConn1 -- Inductor49/RConn1 -- Capacitor25/LConn1
  Inductor54/LConn1 -- Inductor53/RConn1 -- Capacitor27/LConn1
  Inductor10/RConn1 -- Inductor11/LConn1
  Inductor30/RConn1 -- Inductor31/LConn1
  Inductor28/RConn1 -- Inductor29/LConn1
  Inductor12/RConn1 -- Inductor13/LConn1
  Inductor24/LConn1 -- Inductor23/RConn1
  Inductor14/RConn1 -- Inductor15/LConn1
  Inductor38/RConn1 -- Inductor49/LConn1
  Inductor19/RConn1 -- Inductor20/LConn1
  Inductor35/RConn1 -- Inductor37/LConn1
  Inductor25/LConn1 -- Inductor16/RConn1
  Inductor4/RConn1 -- Inductor5/LConn1
  Inductor18/LConn1 -- Inductor17/RConn1
  Inductor39/LConn1 -- Inductor36/RConn1
  Inductor45/RConn1 -- Inductor46/LConn1
  Inductor32/RConn1 -- Inductor42/LConn1
  Inductor41/LConn1 -- Inductor40/RConn1
  Inductor21/RConn1 -- Inductor22/LConn1
  Inductor48/LConn1 -- Inductor47/RConn1
  Inductor6/RConn1 -- Inductor7/LConn1
  Inductor52/RConn1 -- Inductor53/LConn1
  Inductor3/LConn1 -- Inductor2/RConn1
  Inductor26/RConn1 -- Inductor27/LConn1
  Inductor9/LConn1 -- Inductor8/RConn1
  Inductor51/LConn1 -- Inductor50/RConn1
  Inductor34/LConn1 -- Inductor33/RConn1
  Inductor43/RConn1 -- Inductor44/LConn1
  Simulink-PS Converter/RConn1 -- Controlled Current Source/RConn1
  PS-Simulink Converter/LConn1 -- Voltage Sensor/RConn1
  Inductor66/LConn1 -- Capacitor28/LConn1 -- Inductor55/RConn1
  Inductor69/LConn1 -- Capacitor29/LConn1 -- Inductor66/RConn1
  Inductor58/RConn1 -- Capacitor31/LConn1 -- Inductor59/LConn1
  Inductor62/RConn1 -- Capacitor35/LConn1 -- Inductor63/LConn1
  Inductor58/LConn1 -- Capacitor30/LConn1 -- Inductor57/RConn1
  Inductor70/RConn1 -- Capacitor41/LConn1 -- Inductor71/LConn1
  Inductor60/RConn1 -- Capacitor33/LConn1 -- Inductor61/LConn1
  Inductor74/RConn1 -- Capacitor45/LConn1 -- Inductor75/LConn1
  Inductor57/LConn1 -- Capacitor47/LConn1 -- Inductor56/RConn1
  Inductor70/LConn1 -- Capacitor40/LConn1 -- Inductor69/RConn1
  Inductor68/LConn1 -- Capacitor39/LConn1 -- Inductor67/RConn1
  Inductor61/RConn1 -- Capacitor34/LConn1 -- Inductor62/LConn1
  Inductor65/RConn1 -- Capacitor38/LConn1 -- Inductor67/LConn1
  Inductor64/RConn1 -- Capacitor37/LConn1 -- Inductor65/LConn1
  Inductor60/LConn1 -- Capacitor32/LConn1 -- Inductor59/RConn1
  Inductor72/RConn1 -- Capacitor43/LConn1 -- Inductor73/LConn1
  Inductor56/LConn1 -- Capacitor46/LConn1 -- Inductor75/RConn1
  Inductor64/LConn1 -- Capacitor36/LConn1 -- Inductor63/RConn1
  Inductor73/RConn1 -- Capacitor44/LConn1 -- Inductor74/LConn1
  Inductor72/LConn1 -- Capacitor42/LConn1 -- Inductor71/RConn1
  Voltage Sensor/RConn2 -- Controlled Current Source/LConn1 -- Capacitor29/RConn1 -- Capacitor40/RConn1 -- Capacitor41/RConn1 -- Capacitor42/RConn1 -- Capacitor43/RConn1 -- Capacitor44/RConn1 -- Capacitor45/RConn1 -- Capacitor46/RConn1 -- Capacitor47/RConn1 -- Capacitor30/RConn1 -- Capacitor31/RConn1 -- Capacitor32/RConn1 -- Capacitor33/RConn1 -- Capacitor34/RConn1 -- Capacitor35/RConn1 -- Capacitor36/RConn1 -- Capacitor37/RConn1 -- Capacitor39/RConn1 -- Capacitor1/RConn1 -- Capacitor3/RConn1 -- Capacitor4/RConn1 -- Capacitor5/RConn1 -- Capacitor6/RConn1 -- Capacitor7/RConn1 -- Capacitor8/RConn1 -- Capacitor9/RConn1 -- Capacitor10/RConn1 -- Capacitor11/RConn1 -- Capacitor12/RConn1 -- Capacitor13/RConn1 -- Capacitor14/RConn1 -- Capacitor16/RConn1 -- Capacitor17/RConn1 -- Capacitor24/RConn1 -- Capacitor25/RConn1 -- Capacitor27/RConn1 -- Resistor1/RConn1 -- Inductor/RConn1 -- Capacitor26/RConn1 -- Capacitor23/RConn1 -- Capacitor22/RConn1 -- Capacitor21/RConn1 -- Capacitor20/RConn1 -- Capacitor19/RConn1 -- Capacitor18/RConn1 -- Capacitor15/RConn1 -- Capacitor2/RConn1 -- Capacitor38/RConn1 -- Capacitor28/RConn1 -- Capacitor48/RConn1 -- Electrical Reference/LConn1
  Inductor68/RConn1 -- Inductor1/LConn1
  Voltage Sensor/LConn1 -- Controlled Current Source/RConn2 -- Capacitor48/LConn1 -- Inductor76/LConn1 -- Solver Configuration/RConn1
  Inductor76/RConn1 -- Inductor55/LConn1
  Current Sensor/LConn1 -- Inductor54/RConn1
  PS-Simulink Converter1/LConn1 -- Current Sensor/RConn1
